simulink library "INT_Rail_CtlLoopParaMeUn"  (R2016b)
settings: Solver=VariableStepAuto  StartTime=0.0  StopTime=10.0  RelTol=1e-3
settings Model: Creator=Administrator  LastModifiedBy=Administrator

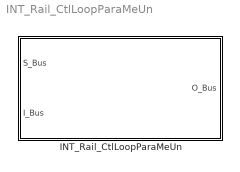
== system INT_Rail_CtlLoopParaMeUn ==
  INT_Rail_CtlLoopParaMeUn : Subsystem

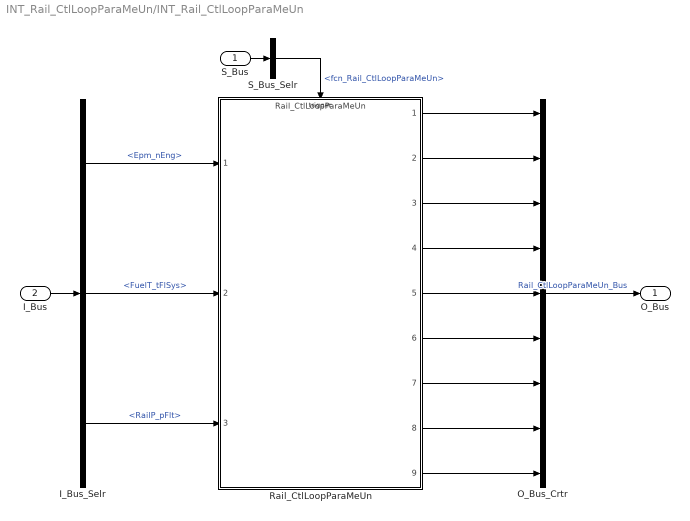
== system INT_Rail_CtlLoopParaMeUn/INT_Rail_CtlLoopParaMeUn ==
  S_Bus : Inport
  I_Bus : Inport  Port=2
  I_Bus_Selr : BusSelector  OutputSignals=Epm_nEng,FuelT_tFlSys,RailP_pFlt
  O_Bus_Crtr : BusCreator  Inputs=9
  Rail_CtlLoopParaMeUn : ModelReference  ModelNameDialog=Rail_CtlLoopParaMeUn  SimulationMode=Normal  ModelReferenceVersion=1.8  TriggerPortName=function  TriggerPortTriggerType=function-call  TriggerPortStatesWhenEnabling=held
  S_Bus_Selr : BusSelector  OutputSignals=fcn_Rail_CtlLoopParaMeUn
  O_Bus : Outport
  wires:
  S_Bus_Selr/1 -> Rail_CtlLoopParaMeUn/Trigger  "<fcn_Rail_CtlLoopParaMeUn>"
  S_Bus/1 -> S_Bus_Selr/1
  I_Bus/1 -> I_Bus_Selr/1
  I_Bus_Selr/1 -> Rail_CtlLoopParaMeUn/1  "<Epm_nEng>"
  I_Bus_Selr/2 -> Rail_CtlLoopParaMeUn/2  "<FuelT_tFlSys>"
  I_Bus_Selr/3 -> Rail_CtlLoopParaMeUn/3  "<RailP_pFlt>"
  O_Bus_Crtr/1 -> O_Bus/1  "Rail_CtlLoopParaMeUn_Bus"
  Rail_CtlLoopParaMeUn/1 -> O_Bus_Crtr/1
  Rail_CtlLoopParaMeUn/2 -> O_Bus_Crtr/2
  Rail_CtlLoopParaMeUn/3 -> O_Bus_Crtr/3
  Rail_CtlLoopParaMeUn/4 -> O_Bus_Crtr/4
  Rail_CtlLoopParaMeUn/5 -> O_Bus_Crtr/5
  Rail_CtlLoopParaMeUn/6 -> O_Bus_Crtr/6
  Rail_CtlLoopParaMeUn/7 -> O_Bus_Crtr/7
  Rail_CtlLoopParaMeUn/8 -> O_Bus_Crtr/8
  Rail_CtlLoopParaMeUn/9 -> O_Bus_Crtr/9
